simulink model "MissionSupervisor_2019a"  (R2019b)
settings: Solver=VariableStepAuto  StartTime=0.0  StopTime=10.0  RelTol=1e-3
undefined symbols (not defined in the file or in its folder): DiscIntNeverNeededParam
libraries: simulink x2
(part 3 of 3)

== matlab function MissionSupervisor_2019a/Mission Supervisor Def/Trasf. to NED ==
  data: posArg input; pos output; areaOfInterestCorner parameter
function pos = LLD2NED(posArg,areaOfInterestCorner)
    coder.extrinsic('evalin','wgs84Ellipsoid','geodetic2ned');
    pos = zeros(1,3);
    pos1 = 0;
    pos2 = 0;
    pos3 = 0;
    [pos1, pos2, pos3] = geodetic2ned(posArg(1), posArg(2), posArg(3),areaOfInterestCorner(1), areaOfInterestCorner(2), 0,wgs84Ellipsoid);
    pos = [pos1, pos2, posArg(3)];
end

== matlab function MissionSupervisor_2019a/Mission Supervisor Def/Trasf. to LLD ==
  data: posArg input; pos output; areaOfInterestCorner parameter
function pos = NED2LLD(posArg,areaOfInterestCorner)
    coder.extrinsic('evalin','wgs84Ellipsoid','ned2geodetic');
    pos = zeros(1,3);
    pos1 = 0;
    pos2 = 0;
    pos3 = 0;
    [pos1, pos2, pos3] = ned2geodetic(posArg(1), posArg(2), posArg(3),areaOfInterestCorner(1), areaOfInterestCorner(2), 0,wgs84Ellipsoid);
    pos = [pos1, pos2, posArg(3)];%-posArg(3)];
end
